simulink model "termic"  (Simulink 7.2)
settings: Solver=ode45  StartTime=0.0  StopTime=7000.0  RelTol=1e-3
undefined symbols (not defined in the file): T
settings Model: Creator=dpara  LastModifiedBy=dpara

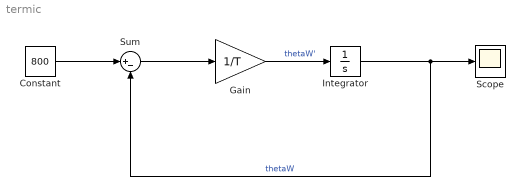
== system termic ==
  Constant : Constant  Value=800  OutDataType=sfix(16)  OutScaling=2^0
  Gain : Gain  Gain=1/T  ParameterDataType=sfix(16)  ParameterScaling=2^0  OutDataType=sfix(16)  OutScaling=2^0
  Integrator : Integrator  InitialCondition=20
  Scope : Scope
  Sum : Sum  Inputs=|+-  OutDataType=sfix(16)  OutScaling=2^0
  wires:
  Constant/1 -> Sum/1
  Sum/1 -> Gain/1
  Integrator/1 -> Sum/2, Scope/1  "thetaW"
  Gain/1 -> Integrator/1  "thetaW'"
